simulink model "AOO_mode_assignment1"  (R2021a)
settings: Solver=FixedStepAuto  StartTime=0.0  StopTime=10.0  FixedStep=1e-3  RelTol=1e-3  EnableMultiTasking=on
undefined symbols (not defined in the file): D10, D11, D12, D2, D4, D5, D7, D8, D9, PTA0, PTA2, PTB23, PTB9, PTC3, PTC4, PTD0, PTD2, PTD3
libraries: frdmk64flib x9
settings Model: ExtModeTrigDuration=5  Creator=majet  LastModifiedBy=majet

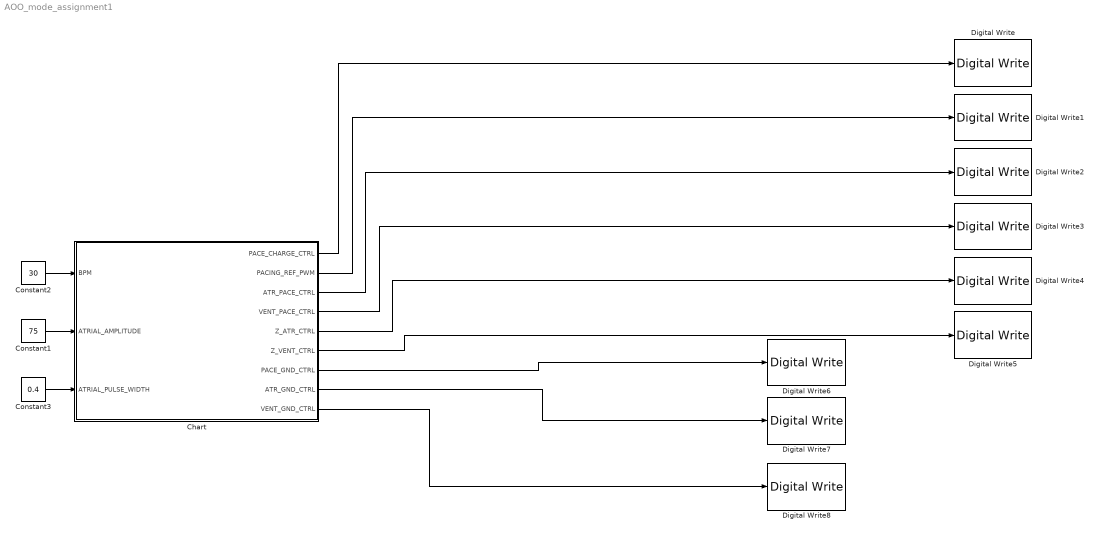
== system AOO_mode_assignment1 ==
  Chart : Stateflow chart  TreatAsAtomicUnit=on
      settings: PortSchema="{\"entries\":[{\"content\":{\"sides\":[{\"content\":{\"connectorIds\":[\"In1\",\"In2\",\"In3\"]},\"type\":\"ConnectorPlacement.EquallySpacedRectSide\",\"uuid\":\"a22e05d8-b46e-41db-a99f-a3bab389e16c\"},{\"content\":{\"connectorIds\":[\"Out3\",\"Out5\",\"Out2\",\"Out7\",\"Out8\",\"Out9\",\"Out4\",\"Out1\",\"Out6\"],\"side\":\"RIGHT\"},\"type\":\"ConnectorPlacement.EquallySpacedRectSide\",\"uuid\":\"b830ec1d-656a-4b92-afcd-8fda6b31ad8a\"},{\"content\":{\"connectorIds\":[],\"side\":\"TOP\"},\"type\":\"ConnectorPlacement.EquallySpacedRectSide\",\"uuid\":\"956e5d71-b4a8-48ca-aae1-84adff4c1ec1\"}]},\"type\":\"ConnectorPlacement.EquallySpacedConnector\",\"uuid\":\"bd48be11-38ec-46b0-b71c-a53820608697\"}],\"packageUris\":[\"http://schema.mathworks.com/mf0/Connector/R2020b\"],\"version\":\"1.0\"}"
  Constant1 : Constant  Value=75
  Constant2 : Constant  Value=30
  Constant3 : Constant  Value=0.4
  Digital Write : frdmk64flib/Digital Write  Whichpin=PTB9 (D2)
  Digital Write1 : frdmk64flib/Digital Write  Whichpin=PTA2 (D5)
  Digital Write2 : frdmk64flib/Digital Write  Whichpin=PTA0 (D8)
  Digital Write3 : frdmk64flib/Digital Write  Whichpin=PTC4 (D9)
  Digital Write4 : frdmk64flib/Digital Write  Whichpin=PTB23 (D4)
  Digital Write5 : frdmk64flib/Digital Write  Whichpin=PTC3 (D7)
  Digital Write6 : frdmk64flib/Digital Write  Whichpin=PTD0 (D10)
  Digital Write7 : frdmk64flib/Digital Write  Whichpin=PTD2 (D11)
  Digital Write8 : frdmk64flib/Digital Write  Whichpin=PTD3 (D12)
  wires:
  Chart/4(PACE_GND_CTRL) -> Digital Write6/1
  Chart/2(ATR_PACE_CTRL) -> Digital Write2/1
  Chart/6(VENT_GND_CTRL) -> Digital Write8/1
  Chart/9(Z_VENT_CTRL) -> Digital Write5/1
  Chart/8(Z_ATR_CTRL) -> Digital Write4/1
  Constant2/1 -> Chart/1(BPM)
  Chart/3(PACE_CHARGE_CTRL) -> Digital Write/1
  Constant1/1 -> Chart/2(ATRIAL_AMPLITUDE)
  Chart/1(ATR_GND_CTRL) -> Digital Write7/1
  Chart/5(PACING_REF_PWM) -> Digital Write1/1
  Chart/7(VENT_PACE_CTRL) -> Digital Write3/1
  Constant3/1 -> Chart/3(ATRIAL_PULSE_WIDTH)

== stateflow chart AOO_mode_assignment1/Chart ==
  state PACE_ATR
    entry:
    PACE_CHARGE_CTRL = 0;
    PACE_GND_CTRL = 1;
    VENT_GND_CTRL = 0;
    VENT_PACE_CTRL = 0;
    Z_ATR_CTRL = 0;
    Z_VENT_CTRL = 0;
    ATR_GND_CTRL = 0;
    ATR_PACE_CTRL = 1;
  state C22_CHARGE
    entry:
    ATR_PACE_CTRL = 0;
    VENT_PACE_CTRL = 0;
    PACING_REF_PWM = ATRIAL_AMPLITUDE;
    PACE_CHARGE_CTRL = 1;
  state C21_DISCHARGE
    entry:
    PACE_GND_CTRL = 1;
    VENT_PACE_CTRL = 0;
    Z_ATR_CTRL = 0;
    Z_VENT_CTRL = 0;
    ATR_PACE_CTRL = 0;
    ATR_GND_CTRL = 1;
    VENT_GND_CTRL = 0;
  (default) -> C22_CHARGE
  C22_CHARGE -> PACE_ATR : after(60/BPM,sec)
  C21_DISCHARGE -> C22_CHARGE
  PACE_ATR -> C21_DISCHARGE : after(ATRIAL_PULSE_WIDTH, msec)
  data: ATR_GND_CTRL output; ATR_PACE_CTRL output; PACE_CHARGE_CTRL output; PACE_GND_CTRL output; PACING_REF_PWM output; VENT_GND_CTRL output; VENT_PACE_CTRL output; BPM input; ATRIAL_AMPLITUDE input; ATRIAL_PULSE_WIDTH input; Z_ATR_CTRL output; Z_VENT_CTRL output
